simulink model "CubeSat_Simulator"  (R2019a)
settings: Solver=ode4  StartTime=0.0  StopTime=54000  FixedStep=0.1  RelTol=1e-5
model workspace: external: MATLAB File C:\Users\Heyang Zhang\OneDrive\02_Education\01_Undergraduate\02_Capstone\Killick-1 CubeSat\05_Technical\01_Simulation\01_Killick1\Simscape\Killick1_simScape_DataFile.m (data not in the file)
values from neighbouring files (symbols this model uses):
  a_desired = 0.35    [CubeSat_Parameter.m]
  D_distri = G_s.'* inv(G_s * G_s.')    [CubeSat_Parameter.m]
  G_s = [-cos(a_inc)*sin(b_rot)  -cos(a_inc)*cos(b_rot)   cos(a_inc)*sin(b_rot)  cos(a_inc)*cos(b_rot) ... (first row only)    [CubeSat_Parameter.m]
  I_rw = I_s - sum_rw    [CubeSat_Parameter.m]
  I_w = [3500E-9  3500E-9  3500E-9  3500E-9 ... (first row only)    [CubeSat_Parameter.m]
  Kc = [eye(3).*[2.5;2.5;2.5]  eye(3).*[5;5;5]]    [CubeSat_Parameter.m]
  Ki = [eye(3).*[1.2 1.2 1.2]  eye(3).*[3;3;3]]    [CubeSat_Parameter.m]
  Kw_d = 0.4    [CubeSat_Parameter.m]
  Kw_i = 0.1    [CubeSat_Parameter.m]
  Kw_p = 0.4    [CubeSat_Parameter.m]
  OMEGA_0 = [0;0;0]    [CubeSat_Parameter.m]
  quat_0 = eul2quat(eulr_0).'    [CubeSat_Parameter.m]
  SatMass = 3.5    [CubeSat_Parameter.m]
  tau_sat_mt = 1e-3    (= 0.001)    [CubeSat_Parameter.m]
  tau_sat_rw = 5e-3    (= 0.005)    [CubeSat_Parameter.m]
  w_desired = 0.35    [CubeSat_Parameter.m]
  w_rw_ref = [0;0;-0;-0]    [CubeSat_Parameter.m]
undefined symbols (not defined in the file or in its folder): Earth, IAU, km, Kp, Kv, s, WGS84
libraries: sharedutil x19, aerolibutil x18, dspmathops x18, sharedtransform x13, simulink_extras x8, aerolibtransform2 x5, simulink x5, asbCubeSatBlockLib x5, aerolibconvert2 x3, dsparch4 x3, ADCS_lib x2, aerolibcelestial x2
(part 1 of 3)
settings Model: Creator=student  LastModifiedBy=Heyang Zhang
settings SolverCC: AlgebraicLoopSolver=LineSearch
settings DataIOCC: ReturnWorkspaceOutputs=off
settings DebuggingCC: AlgebraicLoopMsg=none  ArithmeticOperatorsInVariantConditions=warning
settings SFSimCC: SimUseLocalCustomCode=off
settings RTWCC: RTWUseLocalCustomCode=off

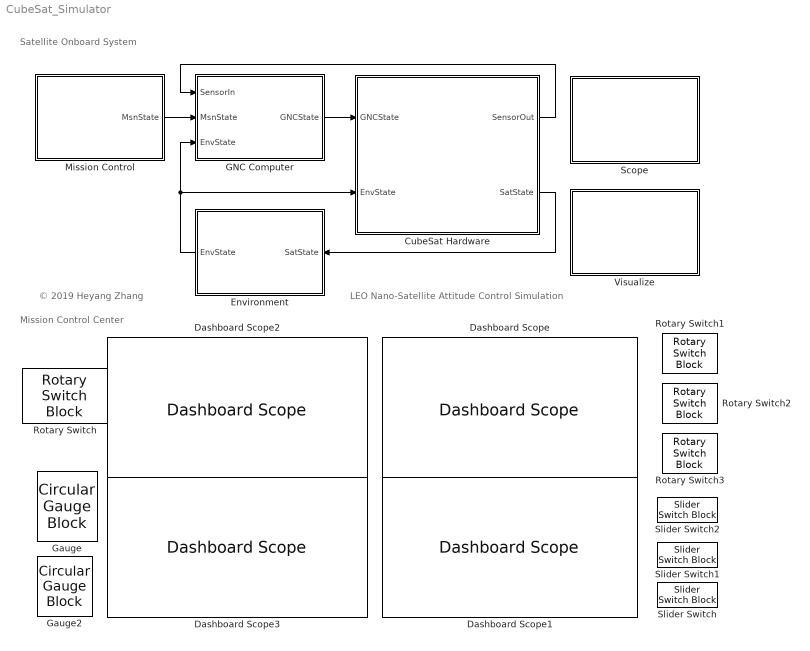
== system CubeSat_Simulator ==
  note: © 2019 Heyang Zhang
  note: LEO Nano-Satellite Attitude Control Simulation
  note: Satellite Onboard System
  note: Mission Control Center
  CubeSat Hardware : Subsystem
  Dashboard Scope{,1..3} (4 alike) : DashboardScope  ShowInitialText=off
  Environment : Subsystem
  GNC Computer : Subsystem
  Gauge : CircularGaugeBlock
  Gauge2 : CircularGaugeBlock
  Mission Control : Subsystem
  Rotary Switch{,1..3} (4 alike) : RotarySwitchBlock  LabelPosition=Bottom
  Scope : Subsystem
  Slider Switch : SliderSwitchBlock  LabelPosition=Bottom
      settings: Values={{'Off', 'On'}, [0 1]}
  Slider Switch1 : SliderSwitchBlock  LabelPosition=Bottom
      settings: Values={{'Off', 'On'}, [0 1]}
  Slider Switch2 : SliderSwitchBlock  LabelPosition=Bottom
      settings: Values={{'Off', 'On'}, [0 1]}
  Visualize : Subsystem
  wires:
  CubeSat Hardware/2(SatState) -> Environment/1(SatState)
  CubeSat Hardware/1(SensorOut) -> GNC Computer/1(SensorIn)
  GNC Computer/1(GNCState) -> CubeSat Hardware/1(GNCState)
  Mission Control/1(MsnState) -> GNC Computer/2(MsnState)
  Environment/1(EnvState) -> GNC Computer/3(EnvState), CubeSat Hardware/2(EnvState)

== system CubeSat_Simulator/CubeSat Hardware ==
  GNCState : Inport
  EnvState : Inport  Port=2
  Attitude Actuator : Subsystem
  Bus Creator : BusCreator  Inputs=2
  Bus Creator2 : BusCreator  Inputs=1
  Orbit Actuator : Constant  Value=[0;0;0]
  Sensor Suit : Subsystem
  Vehicle Dynamics : Subsystem
  SensorOut : Outport
  SatState : Outport  Port=2
  tag scope: EnvState=global, GNCState=global, SatState=global
  wires:
  Bus Creator/1 -> Vehicle Dynamics/1(ActrState)
  GNCState/1 -> [GNCState], Attitude Actuator/2(CtrlCmd)
  EnvState/1 -> Attitude Actuator/3(EnvState), [EnvState], Vehicle Dynamics/2(EnvState)
  Bus Creator2/1 -> Bus Creator/2  "Orbit"
  Vehicle Dynamics/1(SatState) -> SatState/1, Attitude Actuator/1(SatState), Sensor Suit/1(SatState), [SatState]
  Attitude Actuator/1(AttiActr) -> Bus Creator/1  "Attitude"
  Orbit Actuator/1 -> Bus Creator2/1  "CtrlForce"
  Sensor Suit/1(SensorOut) -> SensorOut/1

== system CubeSat_Simulator/Environment ==
  SatState : Inport
  Earth Rotation Planet Position : Subsystem
  External Force and Torque : Subsystem
  Geomagnetic Field : Subsystem
  SimTime : Clock
  Out Bus Element1 : Outport  PortName=EnvState  Element=Torque
  Out Bus Element5 : Outport  PortName=EnvState  Element=Force
  Out Bus Element4 : Outport  PortName=EnvState  Element=Celestrial
  Out Bus Element2 : Outport  PortName=EnvState  Element=Magnetic
  wires:
  External Force and Torque/1(Force) -> Out Bus Element5/1
  Geomagnetic Field/1(Magnetic) -> Out Bus Element2/1
  Earth Rotation Planet Position/1(Celestrial) -> External Force and Torque/2(Celestrial), Geomagnetic Field/2(Celestrial), Out Bus Element4/1
  SatState/1 -> External Force and Torque/1(SatState), Geomagnetic Field/1(SatState)
  External Force and Torque/2(Torque) -> Out Bus Element1/1
  SimTime/1 -> Earth Rotation Planet Position/1(ElaspedTime)

== system CubeSat_Simulator/GNC Computer ==
  SensorIn : Inport
  MsnState : Inport  Port=2
  EnvState : Inport  Port=3
  Bus Creator : BusCreator  Inputs=3
  Control : Subsystem
  Ground1 : Ground
  Guidance : Subsystem
  Navigation : Subsystem
  GNCState : Outport
  wires:
  Navigation/1(NavOut) -> Control/2(NavIn)
  SensorIn/1 -> Guidance/3(SensorIn), Navigation/1(SensorIn)
  EnvState/1 -> Guidance/2(EnvState)
  MsnState/1 -> Guidance/1(MsnState)
  Control/1(CtrlOut) -> Bus Creator/3  "Ctrl"
  Ground1/1 -> Bus Creator/2  "Navi"
  Guidance/1(GdnOut) -> Control/1(GdnIn), Bus Creator/1  "Gdnc"
  Bus Creator/1 -> GNCState/1

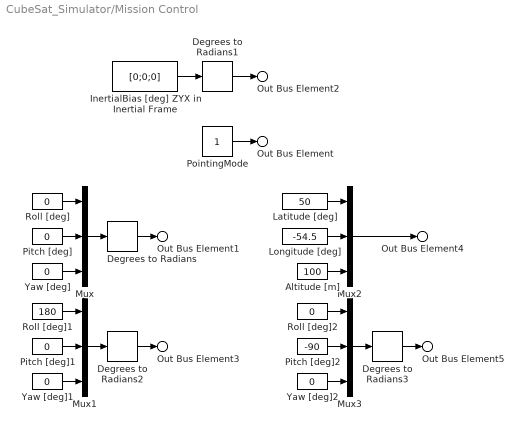
== system CubeSat_Simulator/Mission Control ==
  Altitude [m] : Constant  Value=100
  Degrees to Radians{,1..3} (4 alike) : simulink_extras/Transformations/Degrees to Radians
  InertialBias [deg] ZYX in Inertial Frame : Constant  Value=[0;0;0]
  Latitude [deg] : Constant  Value=50
  Longitude [deg] : Constant  Value=-54.5
  Mux{,1..3} (4 alike) : Mux  Inputs=3
  Pitch [deg] : Constant  Value=0
  Pitch [deg]1 : Constant  Value=0
  Pitch [deg]2 : Constant  Value=-90
  PointingMode : Constant
  Roll [deg] : Constant  Value=0
  Roll [deg]1 : Constant  Value=180
  Roll [deg]2 : Constant  Value=0
  Yaw [deg] : Constant  Value=0
  Yaw [deg]1 : Constant  Value=0
  Yaw [deg]2 : Constant  Value=0
  Out Bus Element : Outport  PortName=MsnState  Element=PointingMode
  Out Bus Element1 : Outport  PortName=MsnState  Element=NadirBias
  Out Bus Element2 : Outport  PortName=MsnState  Element=InertialBias
  Out Bus Element3 : Outport  PortName=MsnState  Element=SunBias
  Out Bus Element4 : Outport  PortName=MsnState  Element=TargetLLA
  Out Bus Element5 : Outport  PortName=MsnState  Element=TargetBias
  wires:
  PointingMode/1 -> Out Bus Element/1
  Degrees to Radians/1 -> Out Bus Element1/1
  Degrees to Radians1/1 -> Out Bus Element2/1
  InertialBias [deg] ZYX in Inertial Frame/1 -> Degrees to Radians1/1
  Mux/1 -> Degrees to Radians/1
  Roll [deg]/1 -> Mux/1
  Pitch [deg]/1 -> Mux/2
  Yaw [deg]/1 -> Mux/3
  Yaw [deg]1/1 -> Mux1/3
  Pitch [deg]1/1 -> Mux1/2
  Roll [deg]1/1 -> Mux1/1
  Mux1/1 -> Degrees to Radians2/1
  Degrees to Radians2/1 -> Out Bus Element3/1
  Longitude [deg]/1 -> Mux2/2
  Altitude [m]/1 -> Mux2/3
  Mux2/1 -> Out Bus Element4/1
  Latitude [deg]/1 -> Mux2/1
  Yaw [deg]2/1 -> Mux3/3
  Pitch [deg]2/1 -> Mux3/2
  Roll [deg]2/1 -> Mux3/1
  Mux3/1 -> Degrees to Radians3/1
  Degrees to Radians3/1 -> Out Bus Element5/1

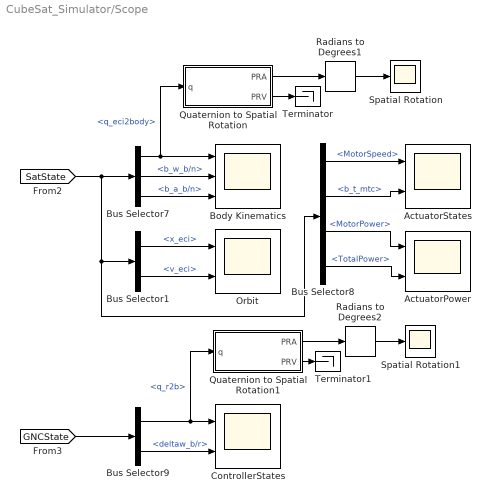
== system CubeSat_Simulator/Scope ==
  ActuatorPower : Scope  NumInputPorts=2
  ActuatorStates : Scope  NumInputPorts=2
  Body Kinematics : Scope  NumInputPorts=3
  Bus Selector1 : BusSelector  OutputSignals=Orbit.x_eci,Orbit.v_eci
  Bus Selector7 : BusSelector  OutputSignals=Attitude.q_eci2body,Attitude.b_w_b/n,Attitude.b_a_b/n
  Bus Selector8 : BusSelector  OutputSignals=Actuator.Attitude.ReactionWheel.MotorSpeed,Actuator.Attitude.MagneticTorquer.b_t_mtc,Actuator.Attitude.ReactionWheel.MotorPower,Actuator.Attitude.ReactionWheel.TotalPower
  Bus Selector9 : BusSelector  OutputSignals=Ctrl.AttitudeCtrl.ACErrData.q_r2b,Ctrl.AttitudeCtrl.ACErrData.deltaw_b/r
  ControllerStates : Scope  NumInputPorts=2
  Orbit : Scope  NumInputPorts=2
  Quaternion to Spatial Rotation : Subsystem
  Quaternion to Spatial Rotation1 : Subsystem
  Radians to Degrees1 : simulink_extras/Transformations/Radians to Degrees
  Radians to Degrees2 : simulink_extras/Transformations/Radians to Degrees
  Spatial Rotation : Scope
  Spatial Rotation1 : Scope
  Terminator : Terminator
  Terminator1 : Terminator
  wires:
  Bus Selector8/1 -> ActuatorStates/1  "<MotorSpeed>"
  Bus Selector8/2 -> ActuatorStates/2  "<b_t_mtc>"
  [GNCState] -> Bus Selector9/1
  [SatState] -> Bus Selector7/1, Bus Selector1/1, Bus Selector8/1
  Bus Selector9/1 -> Quaternion to Spatial Rotation1/1(q), ControllerStates/1  "<q_r2b>"
  Bus Selector8/4 -> ActuatorPower/2  "<TotalPower>"
  Bus Selector7/1 -> Body Kinematics/1, Quaternion to Spatial Rotation/1(q)  "<q_eci2body>"
  Bus Selector7/2 -> Body Kinematics/2  "<b_w_b/n>"
  Bus Selector7/3 -> Body Kinematics/3  "<b_a_b/n>"
  Quaternion to Spatial Rotation/1(PRA) -> Radians to Degrees1/1
  Radians to Degrees1/1 -> Spatial Rotation/1
  Quaternion to Spatial Rotation/2(PRV) -> Terminator/1
  Bus Selector9/2 -> ControllerStates/2  "<deltaw_b/r>"
  Bus Selector1/1 -> Orbit/1  "<x_eci>"
  Bus Selector1/2 -> Orbit/2  "<v_eci>"
  Bus Selector8/3 -> ActuatorPower/1  "<MotorPower>"
  Radians to Degrees2/1 -> Spatial Rotation1/1
  Quaternion to Spatial Rotation1/1(PRA) -> Radians to Degrees2/1
  Quaternion to Spatial Rotation1/2(PRV) -> Terminator1/1

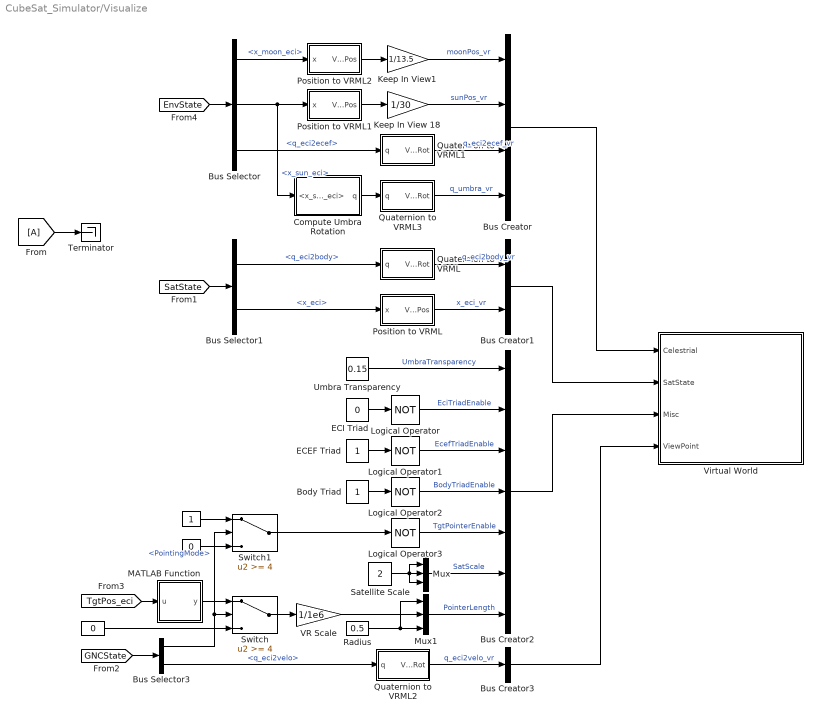
== system CubeSat_Simulator/Visualize ==
  " " : Constant  Value=0
  "  " : Constant  Value=0
  "     " : Constant
  Body Triad : Constant
  Bus Creator : BusCreator  Inputs=4
  Bus Creator1 : BusCreator  Inputs=2
  Bus Creator2 : BusCreator  Inputs=7
  Bus Creator3 : BusCreator  Inputs=1
  Bus Selector : BusSelector  OutputSignals=Celestrial.x_moon_eci,Celestrial.x_sun_eci,Celestrial.q_eci2ecef
  Bus Selector1 : BusSelector  OutputSignals=Attitude.q_eci2body,Orbit.x_eci
  Bus Selector3 : BusSelector  OutputSignals=Gdnc.PointingMode,Gdnc.VrAnim.q_eci2velo
  Compute Umbra Rotation : Subsystem
  ECEF Triad : Constant
  ECI Triad : Constant  Value=0
  Keep In View 18 : Gain  Gain=1/30
  Keep In View1 : Gain  Gain=1/13.5
  Logical Operator{,1..3} (4 alike) : Logic  Operator=NOT  IconShape=distinctive  AllPortsSameDT=off  OutDataTypeStr=boolean
  MATLAB Function : MATLAB Function  TreatAsAtomicUnit=on
  Mux : Mux  Inputs=3
  Mux1 : Mux  Inputs=3
  Position to VRML : Subsystem
  Position to VRML1 : Subsystem
  Position to VRML2 : Subsystem
  Quaternion to VRML : Subsystem
  Quaternion to VRML1 : Subsystem
  Quaternion to VRML2 : Subsystem
  Quaternion to VRML3 : Subsystem
  Radius : Constant  Value=0.5
  Satellite Scale : Constant  Value=2
  Switch : Switch  Threshold=4
  Switch1 : Switch  Threshold=4
  Terminator : Terminator
  Umbra Transparency : Constant  Value=0.15
  VR Scale : Gain  Gain=1/1e6
  Virtual World : Subsystem
  wires:
  Position to VRML/1(VRMLPos) -> Bus Creator1/2  "x_eci_vr"
  Position to VRML1/1(VRMLPos) -> Keep In View 18/1
  Position to VRML2/1(VRMLPos) -> Keep In View1/1
  Keep In View1/1 -> Bus Creator/1  "moonPos_vr"
  Satellite Scale/1 -> Mux/3, Mux/1, Mux/2
  Keep In View 18/1 -> Bus Creator/2  "sunPos_vr"
  Bus Creator/1 -> Virtual World/1(Celestrial)
  Quaternion to VRML1/1(VRMLRot) -> Bus Creator/3  "q_eci2ecef_vr"
  Quaternion to VRML/1(VRMLRot) -> Bus Creator1/1  "q_eci2body_vr"
  Bus Creator1/1 -> Virtual World/2(SatState)
  Mux/1 -> Bus Creator2/6  "SatScale"
  Bus Creator2/1 -> Virtual World/3(Misc)
  ECI Triad/1 -> Logical Operator/1
  ECEF Triad/1 -> Logical Operator1/1
  Body Triad/1 -> Logical Operator2/1
  Logical Operator/1 -> Bus Creator2/2  "EciTriadEnable"
  Logical Operator1/1 -> Bus Creator2/3  "EcefTriadEnable"
  Logical Operator2/1 -> Bus Creator2/4  "BodyTriadEnable"
  [EnvState] -> Bus Selector/1
  Bus Selector/1 -> Position to VRML2/1(x)  "<x_moon_eci>"
  Bus Selector/2 -> Compute Umbra Rotation/1(<x_sun_eci>), Position to VRML1/1(x)  "<x_sun_eci>"
  Bus Selector/3 -> Quaternion to VRML1/1(q)  "<q_eci2ecef>"
  [SatState] -> Bus Selector1/1
  Bus Selector1/2 -> Position to VRML/1(x)  "<x_eci>"
  Bus Selector1/1 -> Quaternion to VRML/1(q)  "<q_eci2body>"
  Bus Creator3/1 -> Virtual World/4(ViewPoint)
  Quaternion to VRML2/1(VRMLRot) -> Bus Creator3/1  "q_eci2velo_vr"
  [GNCState] -> Bus Selector3/1
  Bus Selector3/2 -> Quaternion to VRML2/1(q)  "<q_eci2velo>"
  Switch1/1 -> Logical Operator3/1
  Logical Operator3/1 -> Bus Creator2/5  "TgtPointerEnable"
  Mux1/1 -> Bus Creator2/7  "PointerLength"
  Radius/1 -> Mux1/1, Mux1/3
  VR Scale/1 -> Mux1/2
  Switch/1 -> VR Scale/1
  " "/1 -> Switch/3
  Bus Selector3/1 -> Switch1/2, Switch/2  "<PointingMode>"
  MATLAB Function/1(y) -> Switch/1
  [TgtPos_eci] -> MATLAB Function/1(u)
  "     "/1 -> Switch1/1
  "  "/1 -> Switch1/3
  [A] -> Terminator/1
  Quaternion to VRML3/1(VRMLRot) -> Bus Creator/4  "q_umbra_vr"
  Umbra Transparency/1 -> Bus Creator2/1  "UmbraTransparency"
  Compute Umbra Rotation/1(q) -> Quaternion to VRML3/1(q)

== system CubeSat_Simulator/CubeSat Hardware/Attitude Actuator ==
  In Bus Element4 : Inport  PortName=SatState  Element=Attitude.b_w_b/n
  In Bus Element6 : Inport  PortName=SatState  Element=Attitude.b_a_b/n
  In Bus Element2 : Inport  Port=2  PortName=CtrlCmd  Element=Ctrl.MomentumMgmt.MMTorqCmd.b_t_cmd_rwc
  In Bus Element5 : Inport  Port=2  PortName=CtrlCmd  Element=Ctrl.MomentumMgmt.MMTorqCmd.b_t_cmd_mtc
  In Bus Element3 : Inport  Port=3  PortName=EnvState  Element=Magnetic.B_body
  Bus Creator : BusCreator  Inputs=5
  Bus Creator1 : BusCreator  Inputs=1
  Magnetic Torquer Cluster : Subsystem
  Product : Product
  Reaction Wheel Cluster : Subsystem
  Saturation : Saturate  UpperLimit=tau_sat_rw  LowerLimit=-tau_sat_rw
  Saturation1 : Saturate  UpperLimit=tau_sat_mt  LowerLimit=-tau_sat_mt
  Sum of Elements : Sum  Inputs=+
  Out Bus Element : Outport  PortName=AttiActr  Element=ReactionWheel
  Out Bus Element2 : Outport  PortName=AttiActr  Element=MagneticTorquer
  wires:
  Product/1 -> Sum of Elements/1, Bus Creator/4  "MotorPower"
  In Bus Element4/1 -> Reaction Wheel Cluster/1(b_w_b/n)
  In Bus Element6/1 -> Reaction Wheel Cluster/2(b_a_b/n)
  Reaction Wheel Cluster/2(u_s) -> Bus Creator/2, Product/1  "u_s"
  Magnetic Torquer Cluster/1(t_mtc) -> Bus Creator1/1  "b_t_mtc"
  In Bus Element3/1 -> Magnetic Torquer Cluster/2(Envi)
  Reaction Wheel Cluster/3(omega_w) -> Bus Creator/3, Product/2  "MotorSpeed"
  Saturation/1 -> Reaction Wheel Cluster/3(b_t_cmd_rwc)
  Saturation1/1 -> Magnetic Torquer Cluster/1(b_t_cmd_mtc)
  Reaction Wheel Cluster/1(h_s) -> Bus Creator/1  "h_s"
  Bus Creator/1 -> Out Bus Element/1
  Bus Creator1/1 -> Out Bus Element2/1
  Sum of Elements/1 -> Bus Creator/5  "TotalPower"
  In Bus Element2/1 -> Saturation/1
  In Bus Element5/1 -> Saturation1/1

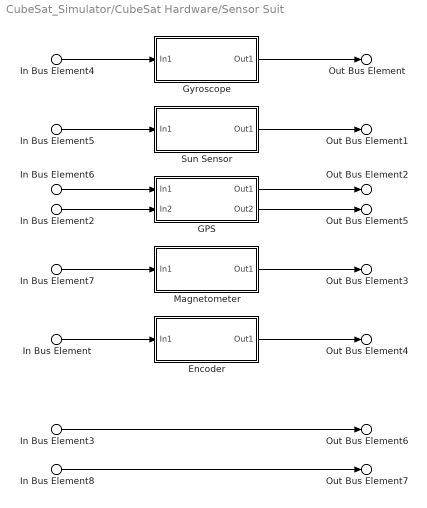
== system CubeSat_Simulator/CubeSat Hardware/Sensor Suit ==
  In Bus Element4 : Inport  PortName=SatState  Element=Attitude.b_w_b/n
  In Bus Element5 : Inport  PortName=SatState  Element=Attitude.q_eci2body
  In Bus Element3 : Inport  PortName=SatState  Element=Attitude.gyroscopic
  In Bus Element8 : Inport  PortName=SatState  Element=Attitude.momentum
  In Bus Element7 : Inport  PortName=SatState  Element=Magnetic.B_body
  In Bus Element : Inport  PortName=SatState  Element=Actuator.Attitude.ReactionWheel.MotorSpeed
  In Bus Element6 : Inport  PortName=SatState  Element=Orbit.x_eci
  In Bus Element2 : Inport  PortName=SatState  Element=Orbit.v_eci
  Encoder : Subsystem
  GPS : Subsystem
  Gyroscope : Subsystem
  Magnetometer : Subsystem
  Sun Sensor : Subsystem
  Out Bus Element : Outport  PortName=SensorOut  Element=b_w_b/n
  Out Bus Element1 : Outport  PortName=SensorOut  Element=q_eci2body
  Out Bus Element2 : Outport  PortName=SensorOut  Element=x_eci
  Out Bus Element3 : Outport  PortName=SensorOut  Element=B_body
  Out Bus Element4 : Outport  PortName=SensorOut  Element=MotorSpeed
  Out Bus Element5 : Outport  PortName=SensorOut  Element=v_eci
  Out Bus Element6 : Outport  PortName=SensorOut  Element=gyroscopic
  Out Bus Element7 : Outport  PortName=SensorOut  Element=momentum
  wires:
  Gyroscope/1(Out1) -> Out Bus Element/1
  Sun Sensor/1(Out1) -> Out Bus Element1/1
  GPS/1(Out1) -> Out Bus Element2/1
  In Bus Element4/1 -> Gyroscope/1(In1)
  In Bus Element5/1 -> Sun Sensor/1(In1)
  In Bus Element6/1 -> GPS/1(In1)
  In Bus Element7/1 -> Magnetometer/1(In1)
  Magnetometer/1(Out1) -> Out Bus Element3/1
  In Bus Element/1 -> Encoder/1(In1)
  Encoder/1(Out1) -> Out Bus Element4/1
  GPS/2(Out2) -> Out Bus Element5/1
  In Bus Element2/1 -> GPS/2(In2)
  In Bus Element3/1 -> Out Bus Element6/1
  In Bus Element8/1 -> Out Bus Element7/1

== system CubeSat_Simulator/CubeSat Hardware/Vehicle Dynamics ==
  In Bus Element3 : Inport  PortName=ActrState
  In Bus Element2 : Inport  PortName=ActrState  Element=Attitude
  In Bus Element6 : Inport  PortName=ActrState  Element=Orbit
  In Bus Element : Inport  Port=2  PortName=EnvState  Element=Force.f_sum_eci
  In Bus Element5 : Inport  Port=2  PortName=EnvState  Element=Torque.t_sum_body
  In Bus Element4 : Inport  Port=2  PortName=EnvState  Element=Magnetic
  Add : Sum  Inputs=|++
  Add1 : Sum  Inputs=|++
  Attitude : Subsystem
  Bus Selector : BusSelector  OutputSignals=ReactionWheel,MagneticTorquer
  Bus Selector1 : BusSelector  OutputSignals=b_t_mtc
  Bus Selector2 : BusSelector  OutputSignals=CtrlForce
  Orbital : Subsystem
  Out Bus Element : Outport  PortName=SatState  Element=Attitude
  Out Bus Element1 : Outport  PortName=SatState  Element=Orbit
  Out Bus Element2 : Outport  PortName=SatState  Element=Actuator
  Out Bus Element3 : Outport  PortName=SatState  Element=Magnetic
  wires:
  Add/1 -> Attitude/2(ExtTorq_body)
  In Bus Element5/1 -> Add/2
  Bus Selector/1 -> Attitude/1(RWRecv)  "<ReactionWheel>"
  Bus Selector2/1 -> Add1/1  "<CtrlForce>"
  Add1/1 -> Orbital/1(ExtForce_eci)
  In Bus Element/1 -> Add1/2
  Attitude/1(SatStateAtti) -> Out Bus Element/1
  Orbital/1(SatStateOrbt) -> Out Bus Element1/1
  In Bus Element2/1 -> Bus Selector/1
  Bus Selector/2 -> Bus Selector1/1  "<MagneticTorquer>"
  Bus Selector1/1 -> Add/1  "<b_t_mtc>"
  In Bus Element6/1 -> Bus Selector2/1
  In Bus Element3/1 -> Out Bus Element2/1
  In Bus Element4/1 -> Out Bus Element3/1

== system CubeSat_Simulator/Environment/Earth Rotation Planet Position ==
  ElaspedTime : Inport
  Celestrial Body Position : Subsystem
  "Earth Rotation " : Subsystem
      mask help:
      | Calculates the quaternion between ECI and ECEF
      |
      | Note: change date in IAU2000 block to simulation start date
  Julian Date Conversion : aerolibconvert2/Julian Date Conversion  year=2019  month=July  day=1  hour=0  min=0  sec=0  modflag=off  deltaT=Sec  errorflag=Error
      settings: SourceProductName=Aerospace Blockset  SourceProductBaseCode=AE
  Out Bus Element : Outport  PortName=Celestrial  Element=q_eci2ecef
  Out Bus Element1 : Outport  PortName=Celestrial  Element=q_ecef2eci
  Out Bus Element2 : Outport  PortName=Celestrial  Element=x_sun_eci
  Out Bus Element3 : Outport  PortName=Celestrial  Element=x_moon_eci
  wires:
  Julian Date Conversion/1 -> Celestrial Body Position/1(JulianDate)
  ElaspedTime/1 -> "Earth Rotation "/1(SimTime), Julian Date Conversion/1
  "Earth Rotation "/1(q_eci2ecef) -> Out Bus Element/1
  "Earth Rotation "/2(q_ecef2eci) -> Out Bus Element1/1
  Celestrial Body Position/1(x_sun_eci) -> Out Bus Element2/1
  Celestrial Body Position/2(x_moon_eci) -> Out Bus Element3/1

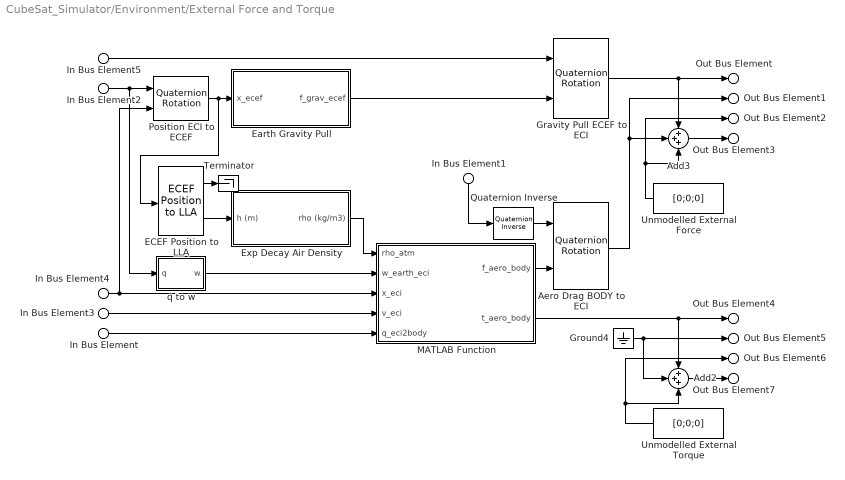
== system CubeSat_Simulator/Environment/External Force and Torque ==
  In Bus Element4 : Inport  PortName=SatState  Element=Orbit.x_eci
  In Bus Element3 : Inport  PortName=SatState  Element=Orbit.v_eci
  In Bus Element : Inport  PortName=SatState  Element=Attitude.q_eci2body
  In Bus Element1 : Inport  PortName=SatState  Element=Attitude.q_eci2body
  In Bus Element2 : Inport  Port=2  PortName=Celestrial  Element=q_eci2ecef
  In Bus Element5 : Inport  Port=2  PortName=Celestrial  Element=q_ecef2eci
  Add2 : Sum  Inputs=+++
  Add3 : Sum  Inputs=+++
  Aero Drag BODY to ECI : aerolibutil/Quaternion Rotation
  ECEF Position to LLA : aerolibtransform2/ECEF Position to LLA  units=Metric (MKS)  ptype=Earth (WGS84)  F=1/298.257223563  R=6378137
      settings: SourceProductName=Aerospace Blockset  SourceProductBaseCode=AE
  Earth Gravity Pull : Subsystem
  Exp Decay Air Density : Subsystem
  Gravity Pull ECEF to ECI : aerolibutil/Quaternion Rotation
  Ground4 : Ground
  MATLAB Function : MATLAB Function  TreatAsAtomicUnit=on  mask{faceNormal=[1 0 0 -1 0 0;0 1 0 0 -1 0;0 0 1 0 0 -1], faceArea=[0.05 0.02 0.01 0.05 0.02 0.01], dragCoeff=[2 2 2 2 2 2], cpLocation=[0.053 0 0 -0.053 0 0;0 0.052 0 0 -0.052 0;0 0 0.112 0 0 -0.112]}
      mask prompts: faceNormal "Facet Normal"; faceArea "Facet Area"; dragCoeff "Drag Coefficient"; cpLocation "CoP Location"
  Position ECI to ECEF : aerolibutil/Quaternion Rotation
  Quaternion Inverse : aerolibutil/Quaternion Inverse
      settings: SourceProductName=Aerospace Blockset
  Terminator : Terminator
  Unmodelled External Force : Constant  Value=[0;0;0]
  Unmodelled External Torque : Constant  Value=[0;0;0]
  q to w : Subsystem
  Out Bus Element : Outport  PortName=Force  Element=f_grav_eci
  Out Bus Element1 : Outport  PortName=Force  Element=f_aero_eci
  Out Bus Element2 : Outport  PortName=Force  Element=f_unmod_eci
  Out Bus Element3 : Outport  PortName=Force  Element=f_sum_eci
  Out Bus Element4 : Outport  Port=2  PortName=Torque  Element=t_aero_body
  Out Bus Element5 : Outport  Port=2  PortName=Torque  Element=t_mag_body
  Out Bus Element6 : Outport  Port=2  PortName=Torque  Element=t_unmod_body
  Out Bus Element7 : Outport  Port=2  PortName=Torque  Element=t_sum_body
  wires:
  Earth Gravity Pull/1(f_grav_ecef) -> Gravity Pull ECEF to ECI/2
  Gravity Pull ECEF to ECI/1 -> Out Bus Element/1, Add3/1
  Unmodelled External Force/1 -> Add3/3, Out Bus Element2/1
  Add3/1 -> Out Bus Element3/1
  In Bus Element5/1 -> Gravity Pull ECEF to ECI/1
  In Bus Element4/1 -> MATLAB Function/3(x_eci), Position ECI to ECEF/2
  q to w/1(w) -> MATLAB Function/2(w_earth_eci)
  In Bus Element2/1 -> Position ECI to ECEF/1, q to w/1(q)
  Position ECI to ECEF/1 -> Earth Gravity Pull/1(x_ecef), ECEF Position to LLA/1
  In Bus Element/1 -> MATLAB Function/5(q_eci2body)
  In Bus Element3/1 -> MATLAB Function/4(v_eci)
  Aero Drag BODY to ECI/1 -> Out Bus Element1/1, Add3/2
  MATLAB Function/1(f_aero_body) -> Aero Drag BODY to ECI/2
  Quaternion Inverse/1 -> Aero Drag BODY to ECI/1
  In Bus Element1/1 -> Quaternion Inverse/1
  Unmodelled External Torque/1 -> Add2/3, Out Bus Element6/1
  Add2/1 -> Out Bus Element7/1
  MATLAB Function/2(t_aero_body) -> Out Bus Element4/1, Add2/1
  Ground4/1 -> Add2/2, Out Bus Element5/1
  ECEF Position to LLA/2 -> Exp Decay Air Density/1(h (m))
  Exp Decay Air Density/1(rho (kg/m3)) -> MATLAB Function/1(rho_atm)
  ECEF Position to LLA/1 -> Terminator/1

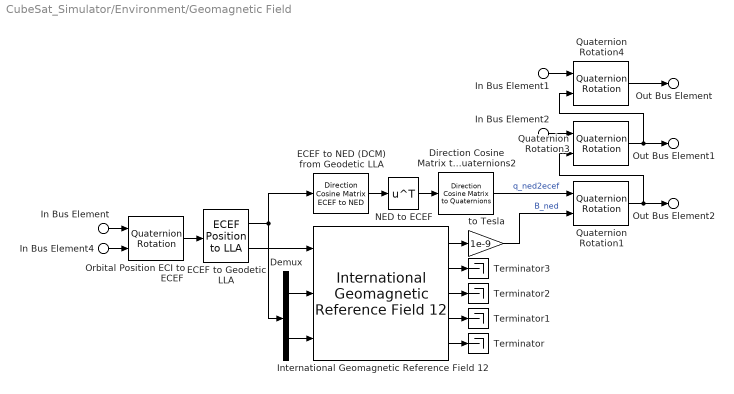
== system CubeSat_Simulator/Environment/Geomagnetic Field ==
  In Bus Element4 : Inport  PortName=SatState  Element=Orbit.x_eci
  In Bus Element1 : Inport  PortName=SatState  Element=Attitude.q_eci2body
  In Bus Element : Inport  Port=2  PortName=Celestrial  Element=q_eci2ecef
  In Bus Element2 : Inport  Port=2  PortName=Celestrial  Element=q_ecef2eci
  Demux : Demux  Outputs=2
  Direction Cosine Matrix to Quaternions2 : sharedtransform/Direction Cosine Matrix  to Quaternions  aMode=0  action=Warning  tolerance=eps(2)
      settings: SourceProductName=Aerospace Blockset  SourceProductBaseCode=AE
  ECEF to Geodetic LLA : aerolibtransform2/ECEF Position to LLA  units=Metric (MKS)  ptype=Earth (WGS84)  F=1/298.257223563  R=6378137
      settings: SourceProductName=Aerospace Blockset  SourceProductBaseCode=AE
  ECEF to NED (DCM) from Geodetic LLA : aerolibtransform2/Direction Cosine Matrix ECEF to NED
      settings: SourceProductName=Aerospace Blockset  SourceProductBaseCode=AE
  "International Geomagnetic Reference Field 12 " : aerolibgravity2/International Geomagnetic Reference Field 12  units=Metric (MKS)  time_in=off  month=January  day=1  year=2019  action=None  sv_out=off
      settings: SourceProductName=Aerospace Blockset  SourceProductBaseCode=AE
  NED to ECEF : Math  Operator=transpose  SaturateOnIntegerOverflow=on
  Orbital Position ECI to ECEF : aerolibutil/Quaternion Rotation
  Quaternion Rotation1 : aerolibutil/Quaternion Rotation
  Quaternion Rotation3 : aerolibutil/Quaternion Rotation
  Quaternion Rotation4 : aerolibutil/Quaternion Rotation
  Terminator{,1..3} (4 alike) : Terminator
  to Tesla : Gain  Gain=1e-9
  Out Bus Element : Outport  PortName=Magnetic  Element=B_body
  Out Bus Element1 : Outport  PortName=Magnetic  Element=B_eci
  Out Bus Element2 : Outport  PortName=Magnetic  Element=B_ecef
  wires:
  Quaternion Rotation3/1 -> Out Bus Element1/1, Quaternion Rotation4/2
  Demux/1 -> "International Geomagnetic Reference Field 12 "/2
  Quaternion Rotation1/1 -> Out Bus Element2/1, Quaternion Rotation3/2
  Direction Cosine Matrix to Quaternions2/1 -> Quaternion Rotation1/1  "q_ned2ecef"
  Demux/2 -> "International Geomagnetic Reference Field 12 "/3
  "International Geomagnetic Reference Field 12 "/1 -> to Tesla/1
  ECEF to Geodetic LLA/1 -> Demux/1, ECEF to NED (DCM) from Geodetic LLA/1
  "International Geomagnetic Reference Field 12 "/5 -> Terminator/1
  ECEF to Geodetic LLA/2 -> "International Geomagnetic Reference Field 12 "/1
  "International Geomagnetic Reference Field 12 "/3 -> Terminator2/1
  ECEF to NED (DCM) from Geodetic LLA/1 -> NED to ECEF/1
  NED to ECEF/1 -> Direction Cosine Matrix to Quaternions2/1
  "International Geomagnetic Reference Field 12 "/2 -> Terminator3/1
  "International Geomagnetic Reference Field 12 "/4 -> Terminator1/1
  Orbital Position ECI to ECEF/1 -> ECEF to Geodetic LLA/1
  In Bus Element1/1 -> Quaternion Rotation4/1
  In Bus Element2/1 -> Quaternion Rotation3/1
  Quaternion Rotation4/1 -> Out Bus Element/1
  to Tesla/1 -> Quaternion Rotation1/2  "B_ned"
  In Bus Element4/1 -> Orbital Position ECI to ECEF/2
  In Bus Element/1 -> Orbital Position ECI to ECEF/1

== system CubeSat_Simulator/GNC Computer/Control ==
  GdnIn : Inport
  NavIn : Inport  Port=2
  Bus Creator : BusCreator  Inputs=2
  Bus Selector1 : BusSelector  OutputSignals=MotorSpeed
  LQI_Full State_Verified : Subsystem  AncestorBlock=ADCS_lib/LQI_Full State_Verified1
      mask help:
      | Gains
      |
      | 1U
      | Kc = [eye(3).*[2.5;2.5;2.5]  eye(3).*[5;5;5]];
      | Ki  = [eye(3).*[1.2 1.2 1.2]  eye(3).*[3;3;3]];
      | Set large Ki velocity gain to surpress oscillation, x & z axis gains have the most effect
      |
      | 3U
  Momentum Management1 : Subsystem
      mask help:
      | Gain
      |
      | 1U
      | Kw_p = 2;
      | Kw_i = 0.2;
      | Kw_d = 0.05;
  PIV Full EoM : Subsystem  Commented=on  AncestorBlock=ADCS_lib/Full EoM Controller
  Out Bus Element : Outport  PortName=CtrlOut  Element=MomentumMgmt
  Out Bus Element1 : Outport  PortName=CtrlOut  Element=AttitudeCtrl
  wires:
  NavIn/1 -> LQI_Full State_Verified/2(NavIn), Bus Selector1/1
  Bus Creator/1 -> Out Bus Element1/1
  Momentum Management1/1(MMCmd) -> Out Bus Element/1
  Bus Selector1/1 -> Momentum Management1/2(w_rw)  "<MotorSpeed>"
  LQI_Full State_Verified/1(ACCmd) -> Momentum Management1/1(ACCmd), Bus Creator/1  "ACTorqCmd"
  LQI_Full State_Verified/2(ErrData) -> Bus Creator/2  "ACErrData"
  GdnIn/1 -> LQI_Full State_Verified/1(GdnIn)

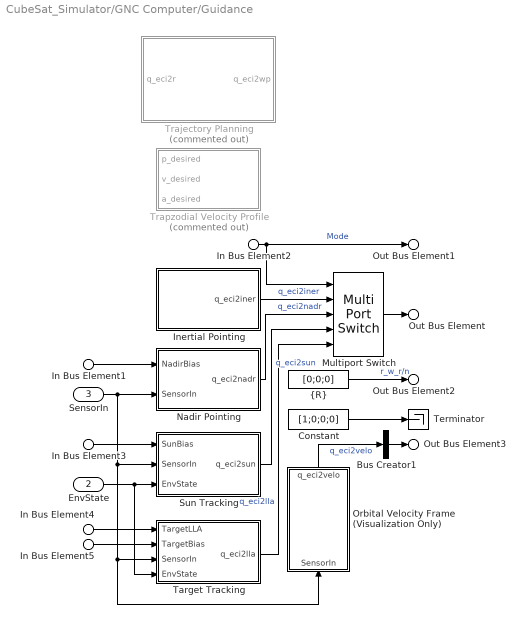
== system CubeSat_Simulator/GNC Computer/Guidance ==
  In Bus Element2 : Inport  PortName=MsnState  Element=PointingMode
  In Bus Element1 : Inport  PortName=MsnState  Element=NadirBias
  In Bus Element3 : Inport  PortName=MsnState  Element=SunBias
  In Bus Element4 : Inport  PortName=MsnState  Element=TargetLLA
  In Bus Element5 : Inport  PortName=MsnState  Element=TargetBias
  EnvState : Inport  Port=2
  SensorIn : Inport  Port=3
  Bus Creator1 : BusCreator  Inputs=1
  Constant : Constant  Value=[1;0;0;0]
  Inertial Pointing : Subsystem
  Multiport Switch : MultiPortSwitch  DataPortOrder=Specify indices  DataPortIndices={1,2,3,4}
  Nadir Pointing : Subsystem
  Orbital Velocity Frame (Visualization Only) : Subsystem
  Sun Tracking : Subsystem
  Target Tracking : Subsystem
  Terminator : Terminator
  Trajectory Planning : Subsystem  Commented=on  AncestorBlock=ADCS_lib/Full EoM Controller
  Trapzodial Velocity Profile : Subsystem  Commented=on
  "{R}" : Constant  Value=[0;0;0]
  Out Bus Element : Outport  PortName=GdnOut  Element=q_eci2ref
  Out Bus Element2 : Outport  PortName=GdnOut  Element=r_w_r/n
  Out Bus Element3 : Outport  PortName=GdnOut  Element=VrAnim
  Out Bus Element1 : Outport  PortName=GdnOut  Element=PointingMode
  wires:
  SensorIn/1 -> Nadir Pointing/2(SensorIn), Sun Tracking/2(SensorIn), Target Tracking/3(SensorIn), Orbital Velocity Frame (Visualization Only)/1(SensorIn)
  In Bus Element1/1 -> Nadir Pointing/1(NadirBias)
  EnvState/1 -> Sun Tracking/3(EnvState), Target Tracking/4(EnvState)
  In Bus Element2/1 -> Multiport Switch/1, Out Bus Element1/1  "Mode"
  Inertial Pointing/1(q_eci2iner) -> Multiport Switch/2  "q_eci2iner"
  Nadir Pointing/1(q_eci2nadr) -> Multiport Switch/3  "q_eci2nadr"
  Sun Tracking/1(q_eci2sun) -> Multiport Switch/4  "q_eci2sun"
  Target Tracking/1(q_eci2lla) -> Multiport Switch/5  "q_eci2lla"
  Orbital Velocity Frame (Visualization Only)/1(q_eci2velo) -> Bus Creator1/1  "q_eci2velo"
  Bus Creator1/1 -> Out Bus Element3/1
  In Bus Element3/1 -> Sun Tracking/1(SunBias)
  In Bus Element4/1 -> Target Tracking/1(TargetLLA)
  In Bus Element5/1 -> Target Tracking/2(TargetBias)
  Multiport Switch/1 -> Out Bus Element/1
  Constant/1 -> Terminator/1
  "{R}"/1 -> Out Bus Element2/1  "r_w_r/n"

== system CubeSat_Simulator/GNC Computer/Navigation ==
  SensorIn : Inport
  NavOut : Outport
  wires:
  SensorIn/1 -> NavOut/1

== system CubeSat_Simulator/Scope/Quaternion to Spatial Rotation ==
  q : Inport
  Constant : Constant  Value=[0;0;0]
  Divide : Product  Inputs=*/
  Gain : Gain  Gain=2
  Normalization : dspmathops/Normalization  NormType=Squared 2-norm  Bias=1e-10  NormOver=Each column  Dimension=1  roundingMode=Floor  overflowMode=off  accumDataTypeStr=Inherit: Same as product output  accumLastDataTypeStr=Inherit: Same as product output  outputDataTypeStr=Inherit: Same as product output  outputMin=[]  outputMax=[]  outputLastDataTypeStr=Inherit: Same as product output
      settings: SourceProductName=DSP System Toolbox
  Resolve Division by 0 : Switch  Criteria=u2 ~= 0
  Scalar Part : Selector  InputPortWidth=4  IndexOptions=Index vector (dialog)  Indices=[1]  OutputSizes=1
  Trigonometric Function : Trigonometry  Operator=acos  OutputSignalType=real
  Trigonometric Function1 : Trigonometry  OutputSignalType=real
  Vector Part : Selector  InputPortWidth=4  IndexOptions=Index vector (dialog)  Indices=[2 3 4]  OutputSizes=1
  PRA : Outport
  PRV : Outport  Port=2
  wires:
  q/1 -> Scalar Part/1, Vector Part/1
  Scalar Part/1 -> Trigonometric Function/1
  Gain/1 -> PRA/1
  Vector Part/1 -> Divide/1
  Trigonometric Function/1 -> Trigonometric Function1/1, Gain/1
  Trigonometric Function1/1 -> Divide/2, Resolve Division by 0/2
  Normalization/1 -> PRV/1
  Divide/1 -> Resolve Division by 0/1
  Resolve Division by 0/1 -> Normalization/1
  Constant/1 -> Resolve Division by 0/3

== system CubeSat_Simulator/Scope/Quaternion to Spatial Rotation1 ==
  q : Inport
  Constant : Constant  Value=[0;0;0]
  Divide : Product  Inputs=*/
  Gain : Gain  Gain=2
  Normalization : dspmathops/Normalization  NormType=Squared 2-norm  Bias=1e-10  NormOver=Each column  Dimension=1  roundingMode=Floor  overflowMode=off  accumDataTypeStr=Inherit: Same as product output  accumLastDataTypeStr=Inherit: Same as product output  outputDataTypeStr=Inherit: Same as product output  outputMin=[]  outputMax=[]  outputLastDataTypeStr=Inherit: Same as product output
      settings: SourceProductName=DSP System Toolbox
  Resolve Division by 0 : Switch  Criteria=u2 ~= 0
  Scalar Part : Selector  InputPortWidth=4  IndexOptions=Index vector (dialog)  Indices=[1]  OutputSizes=1
  Trigonometric Function : Trigonometry  Operator=acos  OutputSignalType=real
  Trigonometric Function1 : Trigonometry  OutputSignalType=real
  Vector Part : Selector  InputPortWidth=4  IndexOptions=Index vector (dialog)  Indices=[2 3 4]  OutputSizes=1
  PRA : Outport
  PRV : Outport  Port=2
  wires:
  Constant/1 -> Resolve Division by 0/3
  Resolve Division by 0/1 -> Normalization/1
  Divide/1 -> Resolve Division by 0/1
  Normalization/1 -> PRV/1
  Trigonometric Function1/1 -> Resolve Division by 0/2, Divide/2
  Trigonometric Function/1 -> Gain/1, Trigonometric Function1/1
  Vector Part/1 -> Divide/1
  Gain/1 -> PRA/1
  Scalar Part/1 -> Trigonometric Function/1
  q/1 -> Vector Part/1, Scalar Part/1

== system CubeSat_Simulator/Visualize/Compute Umbra Rotation ==
  <x_sun_eci> : Inport
  "        " : Constant  Value=[0;0;-1]
  Compute Umbra : asbCubeSatBlockLib/Axes Transformations/Attitude Conversion/Quaternion between r_a and r_b  SystemSampleTime=-1
  Normalization1 : dspmathops/Normalization  NormType=2-norm  Bias=1e-10  NormOver=Each column  Dimension=1  roundingMode=Floor  overflowMode=off  accumDataTypeStr=Inherit: Same as product output  accumLastDataTypeStr=Inherit: Same as product output  outputDataTypeStr=Inherit: Same as product output  outputMin=[]  outputMax=[]  outputLastDataTypeStr=Inherit: Same as product output
      settings: SourceProductName=DSP System Toolbox
  q : Outport
  wires:
  "        "/1 -> Compute Umbra/1
  Compute Umbra/1 -> q/1
  Normalization1/1 -> Compute Umbra/2
  <x_sun_eci>/1 -> Normalization1/1

== system CubeSat_Simulator/Visualize/Position to VRML ==
  x : Inport
  Position to VRML : Selector  InputPortWidth=3  IndexOptions=Index vector (dialog)  Indices=[2 3 1]  OutputSizes=1
  Scale : Gain  Gain=1/1e6
  VRMLPos : Outport
  wires:
  x/1 -> Position to VRML/1
  Position to VRML/1 -> Scale/1
  Scale/1 -> VRMLPos/1

== system CubeSat_Simulator/Visualize/Position to VRML1 ==
  x : Inport
  Position to VRML : Selector  InputPortWidth=3  IndexOptions=Index vector (dialog)  Indices=[2 3 1]  OutputSizes=1
  Scale : Gain  Gain=1/1e6
  VRMLPos : Outport
  wires:
  Scale/1 -> VRMLPos/1
  Position to VRML/1 -> Scale/1
  x/1 -> Position to VRML/1

== system CubeSat_Simulator/Visualize/Position to VRML2 ==
  x : Inport
  Position to VRML : Selector  InputPortWidth=3  IndexOptions=Index vector (dialog)  Indices=[2 3 1]  OutputSizes=1
  Scale : Gain  Gain=1/1e6
  VRMLPos : Outport
  wires:
  x/1 -> Position to VRML/1
  Position to VRML/1 -> Scale/1
  Scale/1 -> VRMLPos/1

== system CubeSat_Simulator/Visualize/Quaternion to VRML ==
  q : Inport
  Constant : Constant  Value=[0;0;0]
  Divide : Product  Inputs=*/
  Gain : Gain  Gain=2
  Mux : Mux  Inputs=2
  Normalization : dspmathops/Normalization  NormType=Squared 2-norm  Bias=1e-10  NormOver=Each column  Dimension=1  roundingMode=Floor  overflowMode=off  accumDataTypeStr=Inherit: Same as product output  accumLastDataTypeStr=Inherit: Same as product output  outputDataTypeStr=Inherit: Same as product output  outputMin=[]  outputMax=[]  outputLastDataTypeStr=Inherit: Same as product output
      settings: SourceProductName=DSP System Toolbox
  Resolve Division by 0 : Switch  Criteria=u2 ~= 0
  Scalar Part : Selector  InputPortWidth=4  IndexOptions=Index vector (dialog)  Indices=[1]  OutputSizes=1
  Selector : Selector  InputPortWidth=4  IndexOptions=Index vector (dialog)  Indices=[3 4 2 1]  OutputSizes=1
  Trigonometric Function : Trigonometry  Operator=acos
  Trigonometric Function1 : Trigonometry  OutputSignalType=real
  Vector Part : Selector  InputPortWidth=4  IndexOptions=Index vector (dialog)  Indices=[2 3 4]  OutputSizes=1
  VRMLRot : Outport
  wires:
  q/1 -> Scalar Part/1, Vector Part/1
  Scalar Part/1 -> Trigonometric Function/1
  Vector Part/1 -> Divide/1
  Trigonometric Function/1 -> Trigonometric Function1/1, Gain/1
  Trigonometric Function1/1 -> Divide/2, Resolve Division by 0/2
  Normalization/1 -> Mux/2
  Divide/1 -> Resolve Division by 0/1
  Resolve Division by 0/1 -> Normalization/1
  Constant/1 -> Resolve Division by 0/3
  Gain/1 -> Mux/1
  Mux/1 -> Selector/1
  Selector/1 -> VRMLRot/1

== system CubeSat_Simulator/Visualize/Quaternion to VRML1 ==
  q : Inport
  Constant : Constant  Value=[0;0;0]
  Divide : Product  Inputs=*/
  Gain : Gain  Gain=2
  Mux : Mux  Inputs=2
  Normalization : dspmathops/Normalization  NormType=Squared 2-norm  Bias=1e-10  NormOver=Each column  Dimension=1  roundingMode=Floor  overflowMode=off  accumDataTypeStr=Inherit: Same as product output  accumLastDataTypeStr=Inherit: Same as product output  outputDataTypeStr=Inherit: Same as product output  outputMin=[]  outputMax=[]  outputLastDataTypeStr=Inherit: Same as product output
      settings: SourceProductName=DSP System Toolbox
  Resolve Division by 0 : Switch  Criteria=u2 ~= 0
  Scalar Part : Selector  InputPortWidth=4  IndexOptions=Index vector (dialog)  Indices=[1]  OutputSizes=1
  Selector : Selector  InputPortWidth=4  IndexOptions=Index vector (dialog)  Indices=[3 4 2 1]  OutputSizes=1
  Trigonometric Function : Trigonometry  Operator=acos
  Trigonometric Function1 : Trigonometry  OutputSignalType=real
  Vector Part : Selector  InputPortWidth=4  IndexOptions=Index vector (dialog)  Indices=[2 3 4]  OutputSizes=1
  VRMLRot : Outport
  wires:
  Selector/1 -> VRMLRot/1
  Mux/1 -> Selector/1
  Gain/1 -> Mux/1
  Constant/1 -> Resolve Division by 0/3
  Resolve Division by 0/1 -> Normalization/1
  Divide/1 -> Resolve Division by 0/1
  Normalization/1 -> Mux/2
  Trigonometric Function1/1 -> Resolve Division by 0/2, Divide/2
  Trigonometric Function/1 -> Gain/1, Trigonometric Function1/1
  Vector Part/1 -> Divide/1
  Scalar Part/1 -> Trigonometric Function/1
  q/1 -> Vector Part/1, Scalar Part/1

== system CubeSat_Simulator/Visualize/Quaternion to VRML2 ==
  q : Inport
  Constant : Constant  Value=[0;0;0]
  Divide : Product  Inputs=*/
  Gain : Gain  Gain=2
  Mux : Mux  Inputs=2
  Normalization : dspmathops/Normalization  NormType=Squared 2-norm  Bias=1e-10  NormOver=Each column  Dimension=1  roundingMode=Floor  overflowMode=off  accumDataTypeStr=Inherit: Same as product output  accumLastDataTypeStr=Inherit: Same as product output  outputDataTypeStr=Inherit: Same as product output  outputMin=[]  outputMax=[]  outputLastDataTypeStr=Inherit: Same as product output
      settings: SourceProductName=DSP System Toolbox
  Resolve Division by 0 : Switch  Criteria=u2 ~= 0
  Scalar Part : Selector  InputPortWidth=4  IndexOptions=Index vector (dialog)  Indices=[1]  OutputSizes=1
  Selector : Selector  InputPortWidth=4  IndexOptions=Index vector (dialog)  Indices=[3 4 2 1]  OutputSizes=1
  Trigonometric Function : Trigonometry  Operator=acos
  Trigonometric Function1 : Trigonometry  OutputSignalType=real
  Vector Part : Selector  InputPortWidth=4  IndexOptions=Index vector (dialog)  Indices=[2 3 4]  OutputSizes=1
  VRMLRot : Outport
  wires:
  Selector/1 -> VRMLRot/1
  Mux/1 -> Selector/1
  Gain/1 -> Mux/1
  Constant/1 -> Resolve Division by 0/3
  Resolve Division by 0/1 -> Normalization/1
  Divide/1 -> Resolve Division by 0/1
  Normalization/1 -> Mux/2
  Trigonometric Function1/1 -> Resolve Division by 0/2, Divide/2
  Trigonometric Function/1 -> Gain/1, Trigonometric Function1/1
  Vector Part/1 -> Divide/1
  Scalar Part/1 -> Trigonometric Function/1
  q/1 -> Vector Part/1, Scalar Part/1

== system CubeSat_Simulator/Visualize/Quaternion to VRML3 ==
  q : Inport
  Constant : Constant  Value=[0;0;0]
  Divide : Product  Inputs=*/
  Gain : Gain  Gain=2
  Mux : Mux  Inputs=2
  Normalization : dspmathops/Normalization  NormType=Squared 2-norm  Bias=1e-10  NormOver=Each column  Dimension=1  roundingMode=Floor  overflowMode=off  accumDataTypeStr=Inherit: Same as product output  accumLastDataTypeStr=Inherit: Same as product output  outputDataTypeStr=Inherit: Same as product output  outputMin=[]  outputMax=[]  outputLastDataTypeStr=Inherit: Same as product output
      settings: SourceProductName=DSP System Toolbox
  Resolve Division by 0 : Switch  Criteria=u2 ~= 0
  Scalar Part : Selector  InputPortWidth=4  IndexOptions=Index vector (dialog)  Indices=[1]  OutputSizes=1
  Selector : Selector  InputPortWidth=4  IndexOptions=Index vector (dialog)  Indices=[3 4 2 1]  OutputSizes=1
  Trigonometric Function : Trigonometry  Operator=acos
  Trigonometric Function1 : Trigonometry  OutputSignalType=real
  Vector Part : Selector  InputPortWidth=4  IndexOptions=Index vector (dialog)  Indices=[2 3 4]  OutputSizes=1
  VRMLRot : Outport
  wires:
  q/1 -> Scalar Part/1, Vector Part/1
  Scalar Part/1 -> Trigonometric Function/1
  Vector Part/1 -> Divide/1
  Trigonometric Function/1 -> Trigonometric Function1/1, Gain/1
  Trigonometric Function1/1 -> Divide/2, Resolve Division by 0/2
  Normalization/1 -> Mux/2
  Divide/1 -> Resolve Division by 0/1
  Resolve Division by 0/1 -> Normalization/1
  Constant/1 -> Resolve Division by 0/3
  Gain/1 -> Mux/1
  Mux/1 -> Selector/1
  Selector/1 -> VRMLRot/1

== system CubeSat_Simulator/Visualize/Virtual World ==
  In Bus Element : Inport  PortName=Celestrial  Element=moonPos_vr
  In Bus Element1 : Inport  PortName=Celestrial  Element=sunPos_vr
  In Bus Element2 : Inport  PortName=Celestrial  Element=q_eci2ecef_vr
  In Bus Element12 : Inport  PortName=Celestrial  Element=q_umbra_vr
  In Bus Element3 : Inport  Port=2  PortName=SatState  Element=q_eci2body_vr
  In Bus Element4 : Inport  Port=2  PortName=SatState  Element=x_eci_vr
  In Bus Element5 : Inport  Port=3  PortName=Misc  Element=SatScale
  In Bus Element6 : Inport  Port=3  PortName=Misc  Element=EciTriadEnable
  In Bus Element7 : Inport  Port=3  PortName=Misc  Element=BodyTriadEnable
  In Bus Element8 : Inport  Port=3  PortName=Misc  Element=EcefTriadEnable
  In Bus Element10 : Inport  Port=3  PortName=Misc  Element=TgtPointerEnable
  In Bus Element11 : Inport  Port=3  PortName=Misc  Element=PointerLength
  In Bus Element13 : Inport  Port=3  PortName=Misc  Element=UmbraTransparency
  In Bus Element9 : Inport  Port=4  PortName=ViewPoint  Element=q_eci2velo_vr
  Satellite Orbit : vrlib/VR Tracer  VrmlFile=C:\Users\Heyang Zhang\OneDrive\02_Education\01_Undergraduate\02_Capstone\Killick-1 CubeSat\05_Technical\01_Simulation\01_Killick1\Visualization\Cubesat_Visualize.wrl  MarkerName=None  UseLines=on  UseTriads=off  MarkerScale=[1 1 1]  MarkerColorSelection=Selected from color list  MarkerColor=white  rgbval=[1 0 0]  Ts=-1  ForceViewerOpen=off  ConnectPlane=off  PlaneCoeff=[0 1 0 0]  ConnectPoint=None  PointCoord=[0 0 0]
      settings: SourceProductName=Simulink  SourceProductBaseCode=SL
  VR Sink (Scale 1e-6) : vrlib/VR Sink  InstantiateOnLoad=on  SampleTime=-1  ViewEnable=on  RemoteChange=off  RemoteView=on  FieldsWritten=Moon.translation.3.1.1.double#Sun.translation.3.1.1.double#Earth.rotation.4.1.1.double#EcefTriadEnable.whichChoice.1.1.1.double#CubeSat.rotation.4.1.1.double#CubeSat.scale.3.1.1.double#CubeSat.translation.3.1.1.double#BodyTriadEnable.whichChoice.1.1.1.double#TargetPointerEnable.whichChoice.1.1.1.double#Pointer.scale.3.1.1.double#EciTriadEnable.whichChoice.1.1.1.double#VeloFrame.rotation.4.1.1.double#VeloFrame.translation.3.1.1.double#Umbra.rotation.4.1.1.double#Transparent.transparency.1.1.1.double  WorldFileName=Visualization\Cubesat_Visualize.wrl  WorldDescription=CubeSat Orbit Visualization  AutoView=on  VideoDimensions=[]  AllowVariableSize=off  FigureProperties="{'Position', 'Name', 'Viewpoint', 'CameraBound', 'CameraDirection', 'CameraPosition', 'CameraUpVector', 'ZoomFactor', 'Antialiasing', 'Headlight', 'Lighting', 'NavPanel', 'Sound', 'StatusBar', 'Stereo3D', 'Stereo3DCameraOffset', 'Stereo3DHIT', 'ToolBar', 'Textures', 'Transparency', 'Triad', 'Wireframe', 'NavZones', 'NavMode', 'NavSpeed', 'CaptureFileFormat', 'CaptureFileName', 'Record2DCompressMethod', 'Record2DCompressQuality', 'Record2D', 'Record2DFileName', 'Record2DFPS'; [8.9900000000000000e+02   1.6900000000000000e+02   7.6600000000000000e+02   6.9100000000000000e+02], 'CubeSat Orbit Visualization', 'Orbital Velocity Follow', 'on', [2.7525454026467437e-02  -4.8175358607383545e-01  -8.7587432413881405e-01], [-1.7620589376263771e-01   3.4875756887157676e+00  -5.3920495462388613e+00], [1.5132242804075643e-02   8.7630672843758750e-01  -4.8151586985552164e-01], [1.0000000000000000e+00], 'on', 'on', 'on', 'halfbar', 'on', 'on', 'off', [1.0000000149011612e-01], [0.0000000000000000e+00], 'on', 'on', 'on', 'none', 'off', 'off', 'examine', 'normal', 'tif', '%f_anim_%n.tif', 'auto', [1.0000000000000000e+02], 'on', 'C:\\Users\\Heyang Zhang\\Desktop\\%f_anim_%n.avi', [6.0000000000000000e+01]}"
      settings: SourceProductName=Simulink
  wires:
  In Bus Element4/1 -> VR Sink (Scale 1e-6)/7, VR Sink (Scale 1e-6)/13, Satellite Orbit/1
  In Bus Element/1 -> VR Sink (Scale 1e-6)/1
  In Bus Element1/1 -> VR Sink (Scale 1e-6)/2
  In Bus Element2/1 -> VR Sink (Scale 1e-6)/3
  In Bus Element8/1 -> VR Sink (Scale 1e-6)/4
  In Bus Element3/1 -> VR Sink (Scale 1e-6)/5
  In Bus Element5/1 -> VR Sink (Scale 1e-6)/6
  In Bus Element7/1 -> VR Sink (Scale 1e-6)/8
  In Bus Element10/1 -> VR Sink (Scale 1e-6)/9
  In Bus Element11/1 -> VR Sink (Scale 1e-6)/10
  In Bus Element6/1 -> VR Sink (Scale 1e-6)/11
  In Bus Element9/1 -> VR Sink (Scale 1e-6)/12
  In Bus Element12/1 -> VR Sink (Scale 1e-6)/14
  In Bus Element13/1 -> VR Sink (Scale 1e-6)/15

== system CubeSat_Simulator/CubeSat Hardware/Attitude Actuator/Magnetic Torquer Cluster ==
  b_t_cmd_mtc : Inport
  Envi : Inport  Port=2
  Terminator : Terminator
  t_mtc : Outport
  wires:
  b_t_cmd_mtc/1 -> t_mtc/1
  Envi/1 -> Terminator/1

== system CubeSat_Simulator/CubeSat Hardware/Attitude Actuator/Reaction Wheel Cluster ==
  b_w_b/n : Inport
  b_a_b/n : Inport  Port=2
  b_t_cmd_rwc : Inport  Port=3
  Demux : Demux
  Distri Mtx2 : Gain  Gain=D_distri  Multiplication=Matrix(K*u)
  Mux1 : Mux
  Mux2 : Mux
  RW 1 : Subsystem
  RW 2 : Subsystem
  RW 3 : Subsystem
  RW 4 : Subsystem
  h_s : Outport
  u_s : Outport  Port=2
  omega_w : Outport  Port=3
  wires:
  Demux/3 -> RW 3/3(u_s_3)
  Demux/1 -> RW 1/3(u_s_1)
  Demux/2 -> RW 2/3(u_s_2)
  Demux/4 -> RW 4/3(u_s_4)
  b_t_cmd_rwc/1 -> Distri Mtx2/1
  b_a_b/n/1 -> RW 1/2(ALPHA), RW 2/2(ALPHA), RW 3/2(ALPHA), RW 4/2(ALPHA)
  RW 1/2(omega_w_1) -> Mux2/1
  Distri Mtx2/1 -> u_s/1, Demux/1  "u_s"
  RW 4/1(h_w_4) -> Mux1/4
  RW 1/1(h_w_1) -> Mux1/1
  Mux2/1 -> omega_w/1
  Mux1/1 -> h_s/1
  RW 3/2(omega_w_3) -> Mux2/3
  RW 4/2(omega_w_4) -> Mux2/4
  b_w_b/n/1 -> RW 4/1(OMEGA), RW 3/1(OMEGA), RW 2/1(OMEGA), RW 1/1(OMEGA)
  RW 3/1(h_w_3) -> Mux1/3
  RW 2/2(omega_w_2) -> Mux2/2
  RW 2/1(h_w_2) -> Mux1/2

== system CubeSat_Simulator/CubeSat Hardware/Sensor Suit/Encoder ==
  In1 : Inport
  Out1 : Outport
  wires:
  In1/1 -> Out1/1

== system CubeSat_Simulator/CubeSat Hardware/Sensor Suit/GPS ==
  In1 : Inport
  In2 : Inport  Port=2
  Out1 : Outport
  Out2 : Outport  Port=2
  wires:
  In1/1 -> Out1/1
  In2/1 -> Out2/1

== system CubeSat_Simulator/CubeSat Hardware/Sensor Suit/Gyroscope ==
  In1 : Inport
  Out1 : Outport
  wires:
  In1/1 -> Out1/1

== system CubeSat_Simulator/CubeSat Hardware/Sensor Suit/Magnetometer ==
  In1 : Inport
  Out1 : Outport
  wires:
  In1/1 -> Out1/1

== system CubeSat_Simulator/CubeSat Hardware/Sensor Suit/Sun Sensor ==
  In1 : Inport
  Out1 : Outport
  wires:
  In1/1 -> Out1/1

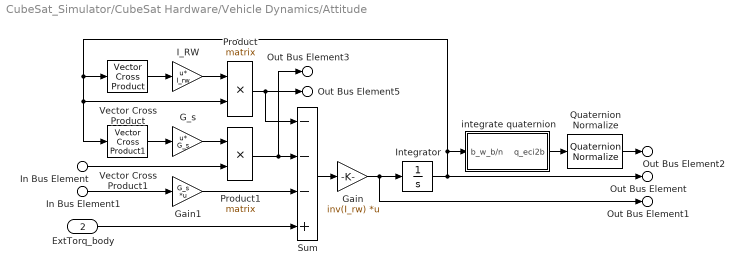
== system CubeSat_Simulator/CubeSat Hardware/Vehicle Dynamics/Attitude ==
  In Bus Element1 : Inport  PortName=RWRecv  Element=u_s
  In Bus Element : Inport  PortName=RWRecv  Element=h_s
  ExtTorq_body : Inport  Port=2
  G_s : Gain  Gain=G_s  Multiplication=Matrix(u*K)
  Gain : Gain  Gain=inv(I_rw)  Multiplication=Matrix(K*u)
  Gain1 : Gain  Gain=G_s  Multiplication=Matrix(K*u)
  I_RW : Gain  Gain=I_rw  Multiplication=Matrix(u*K)
  Integrator : Integrator  InitialCondition=OMEGA_0
  Product : Product  Multiplication=Matrix(*)
  Product1 : Product  Multiplication=Matrix(*)
  Quaternion Normalize : sharedutil/Quaternion Normalize  aMode=aMode
      settings: SourceProductName=Aerospace Blockset  SourceProductBaseCode=AE
  Sum : Sum  Inputs=---+
  Vector Cross Product : ADCS_lib/Dynamics1/Vector Cross Product  SystemSampleTime=-1
  Vector Cross Product1 : ADCS_lib/Dynamics1/Vector Cross Product1  SystemSampleTime=-1
  integrate quaternion : Subsystem  AncestorBlock=ADCS_lib/Dynamics1/integrate quaternion
  Out Bus Element : Outport  PortName=SatStateAtti  Element=b_w_b/n
  Out Bus Element1 : Outport  PortName=SatStateAtti  Element=b_a_b/n
  Out Bus Element2 : Outport  PortName=SatStateAtti  Element=q_eci2body
  Out Bus Element5 : Outport  PortName=SatStateAtti  Element=gyroscopic
  Out Bus Element3 : Outport  PortName=SatStateAtti  Element=momentum
  wires:
  Sum/1 -> Gain/1
  integrate quaternion/1(q_eci2b) -> Quaternion Normalize/1
  Vector Cross Product/1 -> I_RW/1
  I_RW/1 -> Product/1
  Gain/1 -> Integrator/1, Out Bus Element1/1
  Integrator/1 -> Out Bus Element/1, integrate quaternion/1(b_w_b/n), Product/2, Vector Cross Product1/1, Vector Cross Product/1
  In Bus Element/1 -> Product1/2
  Product1/1 -> Sum/2, Out Bus Element3/1
  In Bus Element1/1 -> Gain1/1
  Vector Cross Product1/1 -> G_s/1
  Product/1 -> Sum/1, Out Bus Element5/1
  ExtTorq_body/1 -> Sum/4
  Gain1/1 -> Sum/3
  G_s/1 -> Product1/1
  Quaternion Normalize/1 -> Out Bus Element2/1
